simulink model "Task05"  (R2022b)
settings: Solver=VariableStepAuto  StartTime=0.0  StopTime=10.0  RelTol=1e-3
settings Model: Creator=LOQ  LastModifiedBy=LOQ
settings OptimizationCC: ReuseModelBlockBuffer=on
settings RTWCC: GPUComputeCapability=5.0
settings ConfigComp: CovBoundaryAbsTol=1.0e-5

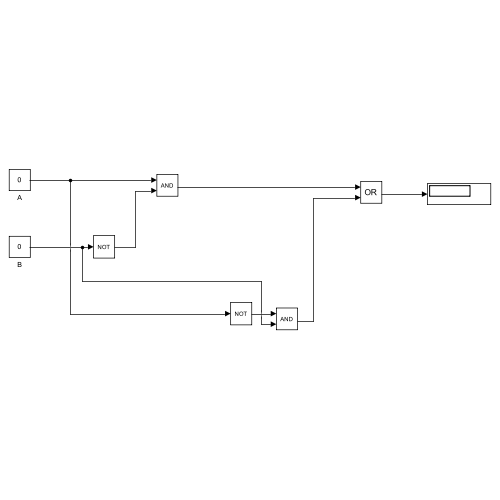
[thumbnail: Simulink's stored preview of the top-level diagram]
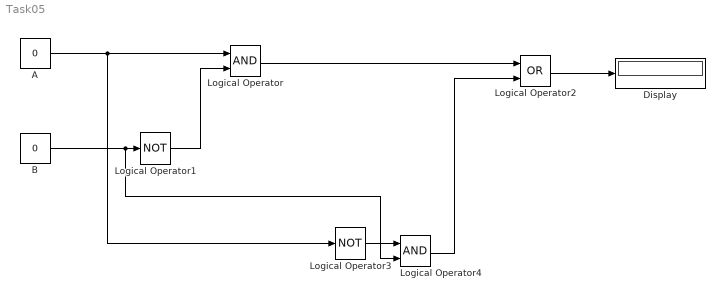
== system Task05 ==
  A : Constant  Value=0
  B : Constant  Value=0
  Display : Display
  Logical Operator : Logic  AllPortsSameDT=off  OutDataTypeStr=boolean
  Logical Operator1 : Logic  Operator=NOT  AllPortsSameDT=off  OutDataTypeStr=boolean
  Logical Operator2 : Logic  Operator=OR  AllPortsSameDT=off  OutDataTypeStr=boolean
  Logical Operator3 : Logic  Operator=NOT  AllPortsSameDT=off  OutDataTypeStr=boolean
  Logical Operator4 : Logic  AllPortsSameDT=off  OutDataTypeStr=boolean
  wires:
  B/1 -> Logical Operator4/2, Logical Operator1/1
  A/1 -> Logical Operator/1, Logical Operator3/1
  Logical Operator1/1 -> Logical Operator/2
  Logical Operator/1 -> Logical Operator2/1
  Logical Operator3/1 -> Logical Operator4/1
  Logical Operator4/1 -> Logical Operator2/2
  Logical Operator2/1 -> Display/1
